simulink model "del1_1_fartsregulering"  (R2024a)
settings: Solver=ode45  StartTime=0.0  StopTime=100  MaxStep=1e-1  MinStep=1e-2  RelTol=1e-1
InitFcn:
  | id_setup()
StopFcn:
  | c_id = evalin('base', "car_id");
  | g_id = evalin('base', "group_id");
  | mqttBasic(c_id,g_id);
  | task = 1.1;
  | score = evalin('base', "score");
  | send_score(task,score);
libraries: init x2, truck_lib x1
settings Model: Creator=adriaeik  LastModifiedBy=adriaeik

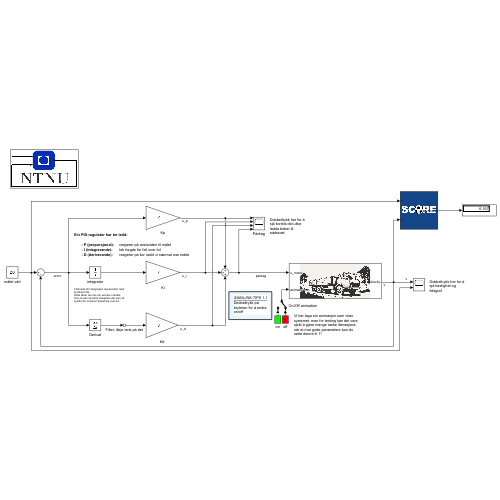
[thumbnail: Simulink's stored preview of the top-level diagram]
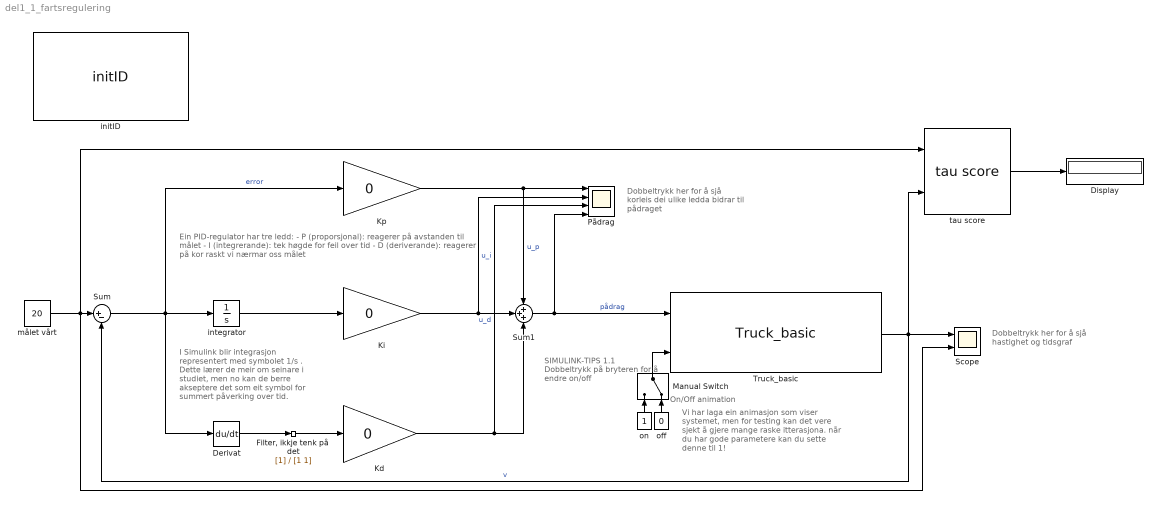
== system del1_1_fartsregulering ==
  note: Dobbeltrykk her for å sjå hastighet og tidsgraf
  note: Vi har laga ein animasjon som viser systemet, men for testing kan det vere sjekt å gjere mange raske itterasjona. når du har gode parametere kan du sette denne til 1!
  note: Ein PID-regulator har tre ledd:
      |
      | - P (proporsjonal): reagerer på avstanden til målet
      | - I (integrerande): tek høgde for feil over tid
      | - D (deriverande): reagerer på kor raskt vi nærmar oss målet
  note: I Simulink blir integrasjon representert med symbolet 1/s .
      | Dette lærer de meir om seinare i studiet, men no kan de berre akseptere det som eit symbol for summert påverking over tid.
  note: On/Off animation
  note: SIMULINK-TIPS 1.1
      | Dobbeltrykk på bryteren for å endre on/off
  note: Dobbeltrykk her for å sjå korleis dei ulike ledda bidrar til pådraget
  Derivat : Derivative
  Display : Display
  "Filter, ikkje tenk på det" : TransferFcn  Denominator=[1 1]
  Kd : Gain  Gain=0
  Ki : Gain  Gain=0
  Kp : Gain  Gain=0
  Manual Switch : ManualSwitch  CurrentSetting=0
  Pådrag : Scope  NumInputPorts=4
  Scope : Scope  NumInputPorts=2
  Sum : Sum  Inputs=|+-
  Sum1 : Sum  Inputs=+++
  Truck_basic : truck_lib/Truck_basic  SystemSampleTime=-1  VariantActivationTime=update diagram  AllowFlexibleInterface=on  Latency=0  AutoFrameSizeCalculation=off
  initID : init/initID  carID=14  groupID=69
  integrator : Integrator
  målet vårt : Constant  Value=20
  off : Constant  Value=0
  on : Constant
  tau score : init/tau score  SystemSampleTime=-1  VariantActivationTime=update diagram  AllowFlexibleInterface=on  Latency=0  AutoFrameSizeCalculation=off
  wires:
  Sum1/1 -> Pådrag/4, Truck_basic/1  "pådrag"
  Truck_basic/1 -> tau score/2, Scope/1, Sum/2  "v"
  Sum/1 -> Kp/1, Derivat/1, integrator/1  "error"
  målet vårt/1 -> tau score/1, Scope/2, Sum/1
  Derivat/1 -> "Filter, ikkje tenk på det"/1
  integrator/1 -> Ki/1
  "Filter, ikkje tenk på det"/1 -> Kd/1
  Ki/1 -> Sum1/2, Pådrag/2  "u_i"
  Kp/1 -> Sum1/1, Pådrag/1  "u_p"
  Kd/1 -> Sum1/3, Pådrag/3  "u_d"
  on/1 -> Manual Switch/1
  Manual Switch/1 -> Truck_basic/2
  off/1 -> Manual Switch/2
  tau score/1 -> Display/1
